simulink model "Compare1Bit"  (R2023a)
settings: Solver=VariableStepAuto  StartTime=0.0  StopTime=1  RelTol=1e-3
settings Model: Creator=Admin  LastModifiedBy=Admin

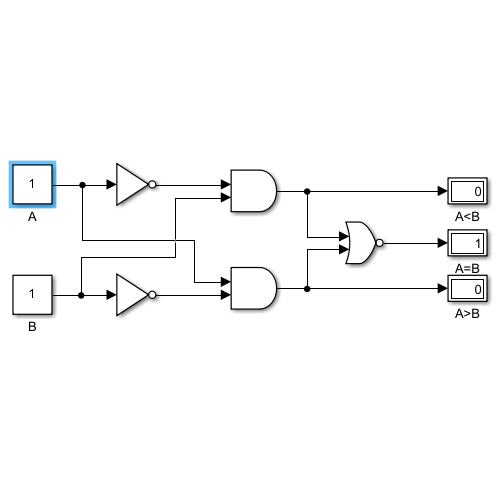
[thumbnail: Simulink's stored preview of the top-level diagram]
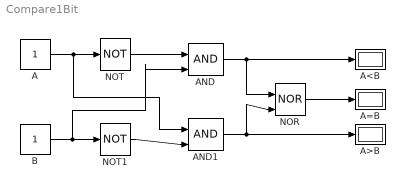
== system Compare1Bit ==
  A : Constant  SampleTime=-1
  A<B : Display
  A=B : Display
  A>B : Display
  AND : Logic  IconShape=distinctive  AllPortsSameDT=off  OutDataTypeStr=boolean
  AND1 : Logic  IconShape=distinctive  AllPortsSameDT=off  OutDataTypeStr=boolean
  B : Constant  SampleTime=-1
  NOR : Logic  Operator=NOR  IconShape=distinctive  AllPortsSameDT=off  OutDataTypeStr=boolean
  NOT : Logic  Operator=NOT  IconShape=distinctive  AllPortsSameDT=off  OutDataTypeStr=boolean
  NOT1 : Logic  Operator=NOT  IconShape=distinctive  AllPortsSameDT=off  OutDataTypeStr=boolean
  wires:
  A/1 -> AND1/1, NOT/1
  NOT/1 -> AND/1
  AND/1 -> A<B/1, NOR/1
  B/1 -> AND/2, NOT1/1
  NOT1/1 -> AND1/2
  NOR/1 -> A=B/1
  AND1/1 -> NOR/2, A>B/1
